simulink model "Actuator_Dynamics"  (R2019b)
settings: Solver=ode4  StartTime=Aircraft_Data.t_i  StopTime=Aircraft_Data.t_f  FixedStep=Aircraft_Data.dt  RelTol=1e-3
PostLoadFcn:
  | %% Adding File Path to MATLAb's Search Path
  | addpath(fileparts(which(bdroot)))
  | 
  | %% Aircraft Data
  | Data_From_Excel = readmatrix('B-747 Flight Condition 5.xlsx','Range','B2:B61');
  | Aircraft_Data = AircraftData(Data_From_Excel);
  | 
  | %% Actuators
  | Servo = tf(10,[1 10]);
  | Engine_TimeLag = tf(0.1,[1 0.1]);
InitFcn:
  | %% Adding File Path to MATLAb's Search Path
  | addpath(fileparts(which(bdroot)))
  | 
  | %% Aircraft Data
  | Data_From_Excel = readmatrix('B-747 Flight Condition 5.xlsx','Range','B2:B61');
  | Aircraft_Data = AircraftData(Data_From_Excel);
  | 
  | %% Actuators
  | Servo = tf(10,[1 10]);
  | Engine_TimeLag = tf(0.1,[1 0.1]);
undefined symbols (not defined in the file or in its folder): theta_0, u_0, w_0
libraries: cstblocks x5
settings Model: Creator=Mahmoud A. Moustafa  LastModifiedBy=Mahmoud A. Moustafa

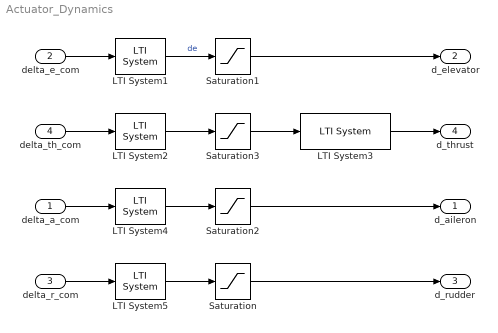
== system Actuator_Dynamics ==
  delta_a_com : Inport
  delta_e_com : Inport  Port=2
  delta_r_com : Inport  Port=3
  delta_th_com : Inport  Port=4
  LTI System1 : cstblocks/LTI System  sys=-Servo  IC=[u_0, w_0, 0, theta_0, 0, 0]
  LTI System2 : cstblocks/LTI System  sys=Servo  IC=[u_0, w_0, 0, theta_0, 0, 0]
  LTI System3 : cstblocks/LTI System  sys=Engine_TimeLag  IC=[u_0, w_0, 0, theta_0, 0, 0]
  LTI System4 : cstblocks/LTI System  sys=Servo  IC=[u_0, w_0, 0, theta_0, 0, 0]
  LTI System5 : cstblocks/LTI System  sys=Servo  IC=[u_0, w_0, 0, theta_0, 0, 0]
  Saturation : Saturate  UpperLimit=25*pi/180  LowerLimit=-25*pi/180
  Saturation1 : Saturate  UpperLimit=25*pi/180  LowerLimit=-25*pi/180
  Saturation2 : Saturate  UpperLimit=25*pi/180  LowerLimit=-25*pi/180
  Saturation3 : Saturate  UpperLimit=47000  LowerLimit=-47000*4*0.75
  d_aileron : Outport
  d_elevator : Outport  Port=2
  d_rudder : Outport  Port=3
  d_thrust : Outport  Port=4
  wires:
  LTI System5/1 -> Saturation/1
  Saturation3/1 -> LTI System3/1
  LTI System1/1 -> Saturation1/1  "de"
  delta_th_com/1 -> LTI System2/1
  LTI System2/1 -> Saturation3/1
  delta_e_com/1 -> LTI System1/1
  Saturation/1 -> d_rudder/1
  Saturation1/1 -> d_elevator/1
  delta_r_com/1 -> LTI System5/1
  LTI System3/1 -> d_thrust/1
  LTI System4/1 -> Saturation2/1
  Saturation2/1 -> d_aileron/1
  delta_a_com/1 -> LTI System4/1
